simulink model "TestCompressor"  (R2019b)
settings: Solver=ode45  StartTime=0.0  StopTime=10.0  RelTol=1e-3  EnableMultiTasking=on
libraries: Lib_TurboC_FlowStart_TMATSC x1, Lib_TurboC_Compressor_TMATSC x1
settings Model: Creator=tlavelle  LastModifiedBy=bhisma
settings DataIOCC: LimitDataPoints=on  SaveFormat=Array  ReturnWorkspaceOutputs=off
settings OptimizationCC: ExpressionDepthLimit=2147483647  LifeSpan=inf
settings DebuggingCC: UnderspecifiedInitializationDetection=Classic  MergeDetectMultiDrivingBlocksExec=none  SolverPrmCheckMsg=warning  StateNameClashWarn=warning  SFUnexpectedBacktrackingDiag=warning  SFNoUnconditionalDefaultTransitionDiag=warning  SFExecutionAtInitializationDiag=none  ArithmeticOperatorsInVariantConditions=warning
settings HardwareCC: ProdBitPerPointer=32  ProdBitPerSizeT=32  ProdBitPerPtrDiffT=32  ProdLargestAtomicFloat=None  ProdIntDivRoundTo=Undefined  ProdEndianess=Unspecified  ProdWordSize=32  ProdHWDeviceType=32-bit Generic
settings ModelReferenceCC: PropagateSignalLabelsOutOfModel=off
settings SFSimCC: SimUseLocalCustomCode=off  CustomCodeUndefinedFunction=UseInterfaceOnly
settings RTWCC: RTWUseLocalCustomCode=off
settings CodeAppCC: StateflowObjectComments=on
settings GRTTargetCC: TargetLangStandard=C89/C90 (ANSI)  GeneratePreprocessorConditionals=Disable all
settings ConfigComp: CovMetricSettings=dw  CovHtmlReporting=on  CovSaveCumulativeToWorkspaceVar=on  CovSaveSingleToWorkspaceVar=on  CovExternalEMLEnable=off

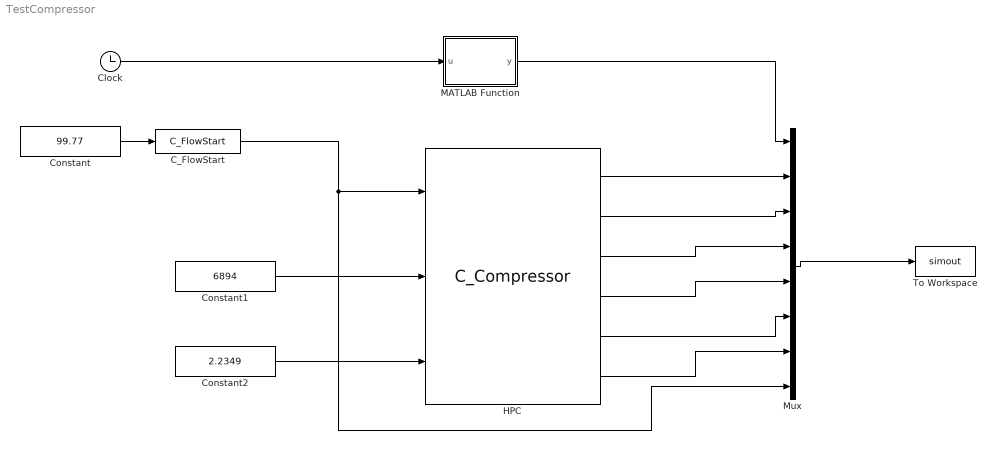
== system TestCompressor ==
  C_FlowStart : Lib_TurboC_FlowStart_TMATSC/C_FlowStart  Tt_M=651.82  Pt_M=21.48  comp1_M=1  comp2_M=0  comp3_M=0  comp4_M=0  comp5_M=0  comp6_M=0
  Clock : Clock
  Constant : Constant  Value=99.77
  Constant1 : Constant  Value=6894
  Constant2 : Constant  Value=2.2349
  HPC : Lib_TurboC_Compressor_TMATSC/C_Compressor  MapFile_M='HPC.map'  s_C_Nc_in_M=.0157  s_Wc_in_M=.4206  s_PR_in_M=.2163  s_eff_in_M=1.0137  Wfrac1_M=.055  hfrac1_M=1  Pfrac1_M=1  Wfrac2_M=.035  hfrac2_M=1  Pfrac2_M=1  IDes_M=2  NcDes_M=100  effDes_M=.8625  PRdes_M=5.679  RlineDes_M=2.0805
  MATLAB Function : MATLAB Function  TreatAsAtomicUnit=on
  Mux : Mux  Inputs=8
  To Workspace : ToWorkspace  VariableName=simout  SaveFormat=Timeseries  SampleTime=-1
  wires:
  C_FlowStart/1 -> HPC/1, Mux/8
  Constant1/1 -> HPC/2
  Constant2/1 -> HPC/3
  Constant/1 -> C_FlowStart/1
  HPC/1 -> Mux/2
  HPC/2 -> Mux/3
  HPC/3 -> Mux/4
  HPC/4 -> Mux/5
  HPC/5 -> Mux/6
  Clock/1 -> MATLAB Function/1(u)
  HPC/6 -> Mux/7
  MATLAB Function/1(y) -> Mux/1
  Mux/1 -> To Workspace/1

== matlab function TestCompressor/MATLAB Function ==
  data: u input; y output
function y = fcn(u)
%#codegen
eml.extrinsic('set_param');
if u < 3
   set_param('TestCompressor/HPC','IDes_M','0');
elseif u< 6 
   set_param('TestCompressor/HPC','IDes_M','1'); 
else 
   set_param('TestCompressor/HPC','IDes_M','2'); 
end    
y = u;
